simulink model "MasodikFeladat"  (R2018b)
settings: Solver=VariableStepAuto  StartTime=0.0  StopTime=8.0  RelTol=1e-3
values from neighbouring files (symbols this model uses):
  A = [0 1; 0 -nu/M]    [LQR.m]    (also in LQR_2feladat.m = [0 1 0; 0 0 -omega^2; 0 1 -1/tau]; LQR_sik.m = [0 1 0 0)
  B = [0 ; 1/M]    [LQR.m]    (also in LQR_2feladat.m = [0 omega^2 0]'; LQR_sik.m = [0 0)
  C = [ 1 0]    [LQR.m]    (also in LQR_2feladat.m = [1 0 0]; LQR_sik.m = [1 0 0 0)
  K1 = R^-1*B'*P    [LQR_2feladat.m]
  x0 = [-2;20]    [LQR.m]    (also in LQR_2feladat.m = [15, 4, 8]; LQR_sik.m = [100; 20; 50; 20])
settings Model: Creator=brajm  LastModifiedBy=brajm

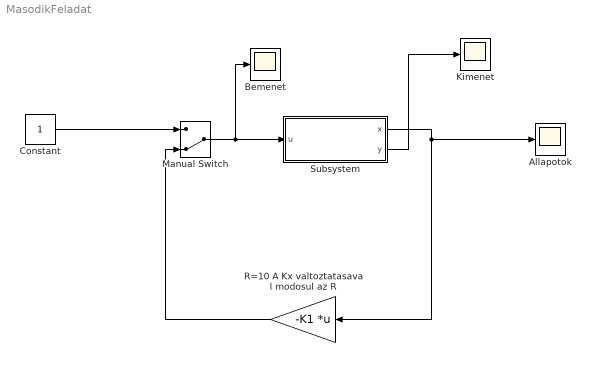
== system MasodikFeladat ==
  "Allapotok " : Scope
  "Bemenet " : Scope
  Constant : Constant
  Kimenet : Scope
  Manual Switch : ManualSwitch  CurrentSetting=0
  "R=10 A Kx valtoztatasaval modosul az R " : Gain  Gain=-K1  Multiplication=Matrix(K*u)
  Subsystem : Subsystem
  wires:
  Manual Switch/1 -> "Bemenet "/1, Subsystem/1(u)
  Subsystem/1(x) -> "R=10 A Kx valtoztatasaval modosul az R "/1, "Allapotok "/1
  "R=10 A Kx valtoztatasaval modosul az R "/1 -> Manual Switch/2
  Subsystem/2(y) -> Kimenet/1
  Constant/1 -> Manual Switch/1

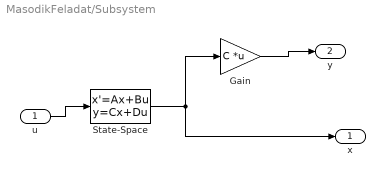
== system MasodikFeladat/Subsystem ==
  u : Inport
  Gain : Gain  Gain=C  Multiplication=Matrix(K*u)
  State-Space : StateSpace  A=A  B=B  C=eye(3)  D=zeros(3,1)  InitialCondition=x0
  x : Outport
  y : Outport  Port=2
  wires:
  u/1 -> State-Space/1
  State-Space/1 -> x/1, Gain/1
  Gain/1 -> y/1
